simulink model "Teensy41_DC_motor_SysId"  (R2025b)
settings: Solver=FixedStepAuto  StartTime=0.0  StopTime=12  RelTol=1e-3  EnableMultiTasking=on
InitFcn:
  | run('Teensy41_system_init.m');
StopFcn:
  | run('Teensy41_to_save_data.m');
values from neighbouring files (symbols this model uses):
  ts = time(2)    [DC_Motor_SysId.m]    (also in DC_Motor_SysId_solve.m)
libraries: arduinolib x22
settings Model: ExtModeTrigDuration=2  Creator=ricardoaguilera  LastModifiedBy=nathan
settings SolverCC: AutoInsertRateTranBlk=on
settings OptimizationCC: EnhancedBackFolding=on  PassReuseOutputArgsAs=Individual arguments  ZeroExternalMemoryAtStartup=off  ZeroInternalMemoryAtStartup=off  MaxStackSize=64  OptimizeBlockOrder=speed  DifferentSizesBufferReuse=on  OptimizationCustomize=off  EfficientTunableParamExpr=on
settings DebuggingCC: ParameterTunabilityLossMsg=error
settings HardwareCC: ProdBitPerPointer=32.0  ProdBitPerSizeT=32.0  ProdBitPerPtrDiffT=32.0  ProdLargestAtomicInteger=Long  ProdLargestAtomicFloat=Double  ProdWordSize=32.0  ProdHWDeviceType=ARM Compatible->ARM Cortex
settings SFSimCC: MATLABDynamicMemAlloc=off
settings RTWCC: SystemTargetFile=ert.tlc  HardwareBoard=Teensy 4.1 (Arduino Compatible)  TemplateMakefile=ert_default_tmf  Toolchain=Arduino ARM M7  BuildConfiguration=Faster Runs  Description=Embedded Coder
settings CodeAppCC: ForceParamTrailComments=on  IgnoreCustomStorageClasses=off  OperatorAnnotations=on  SimulinkDataObjDesc=on  SFDataObjDesc=on  InsertBlockDesc=on
settings ERTTargetCC: ExtModeTransport=3.0  ExtModeStaticAlloc=on  ExtModeAutomaticAllocSize=off  ExtModeStaticAllocSize=65536.0  ExtModeMexFile=ext_xcp  ExtModeIntrfLevel=Level2 - Open  InlinedParameterPlacement=Hierarchical  SupportContinuousTime=on  SupportVariableSizeSignals=on

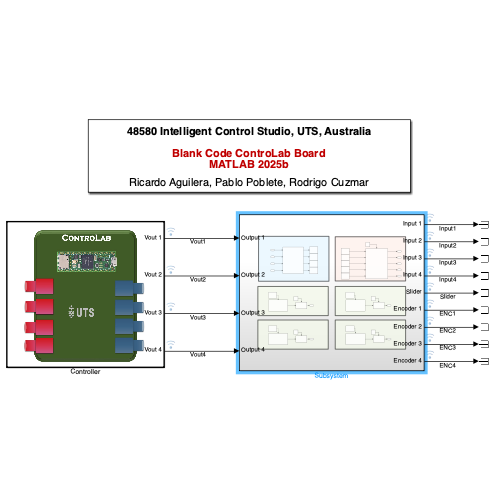
[thumbnail: Simulink's stored preview of the top-level diagram]
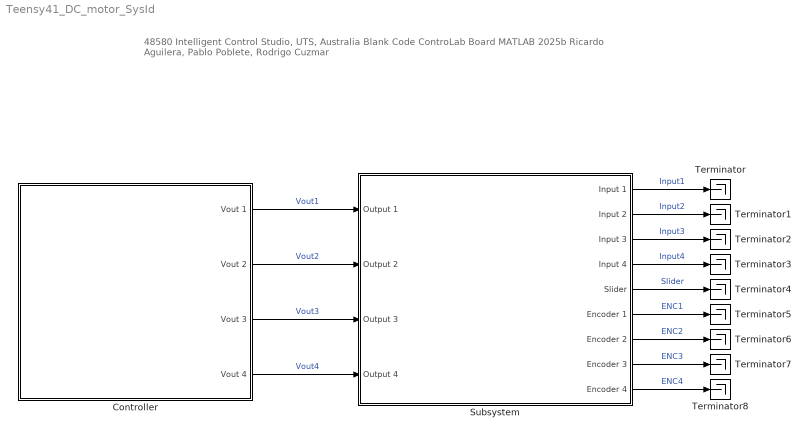
== system Teensy41_DC_motor_SysId ==
  note: 48580 Intelligent Control Studio, UTS, Australia
      |
      | Blank Code ControLab Board
      | MATLAB 2025b
      |
      | Ricardo Aguilera, Pablo Poblete, Rodrigo Cuzmar
  Controller : Subsystem  TreatAsAtomicUnit=on
      mask Display: image('Board_1.png');
  Subsystem : Subsystem
  Terminator{,1..8} (9 alike) : Terminator
  wires:
  Subsystem/8(Encoder 3) -> Terminator7/1  "ENC3"
  Subsystem/7(Encoder 2) -> Terminator6/1  "ENC2"
  Controller/3(Vout 3) -> Subsystem/3(Output 3)  "Vout3"
  Controller/4(Vout 4) -> Subsystem/4(Output 4)  "Vout4"
  Controller/2(Vout 2) -> Subsystem/2(Output 2)  "Vout2"
  Subsystem/5(Slider) -> Terminator4/1  "Slider"
  Subsystem/1(Input 1) -> Terminator/1  "Input1"
  Subsystem/9(Encoder 4) -> Terminator8/1  "ENC4"
  Subsystem/4(Input 4) -> Terminator3/1  "Input4"
  Subsystem/2(Input 2) -> Terminator1/1  "Input2"
  Subsystem/3(Input 3) -> Terminator2/1  "Input3"
  Subsystem/6(Encoder 1) -> Terminator5/1  "ENC1"
  Controller/1(Vout 1) -> Subsystem/1(Output 1)  "Vout1"

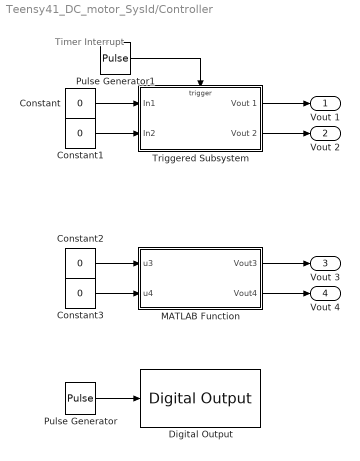
== system Teensy41_DC_motor_SysId/Controller ==
  note: Timer
      | Interrupt
  Constant{,1..3} (4 alike) : Constant  Value=0
  Digital Output : arduinolib/Digital Output  pinNumber=13  Direction=output  blockPlatform=arduino
  MATLAB Function : MATLAB Function  TreatAsAtomicUnit=on  SystemSampleTime=ts
  Pulse Generator : DiscretePulseGenerator  PulseType=Time based  Period=4  PulseWidth=50
  Pulse Generator1 : DiscretePulseGenerator  PulseType=Time based  Period=ts  PulseWidth=50
  Triggered Subsystem : Subsystem  TreatAsAtomicUnit=on
  Vout 1 : Outport
  Vout 2 : Outport  Port=2
  Vout 3 : Outport  Port=3
  Vout 4 : Outport  Port=4
  wires:
  Pulse Generator/1 -> Digital Output/1
  Triggered Subsystem/1(Vout 1) -> Vout 1/1
  Pulse Generator1/1 -> Triggered Subsystem/Trigger
  Constant/1 -> Triggered Subsystem/1(In1)
  MATLAB Function/2(Vout4) -> Vout 4/1
  MATLAB Function/1(Vout3) -> Vout 3/1
  Triggered Subsystem/2(Vout 2) -> Vout 2/1
  Constant1/1 -> Triggered Subsystem/2(In2)
  Constant2/1 -> MATLAB Function/1(u3)
  Constant3/1 -> MATLAB Function/2(u4)

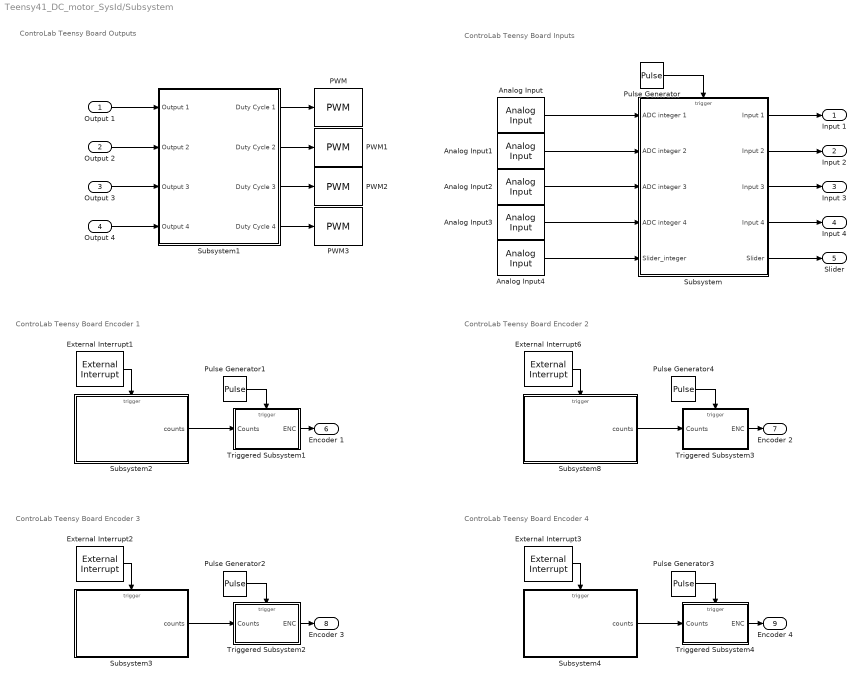
== system Teensy41_DC_motor_SysId/Subsystem ==
  note: ControLab Teensy Board Outputs
  note: ControLab Teensy Board Inputs
  note: ControLab Teensy Board Encoder 2
  note: ControLab Teensy Board Encoder 1
  note: ControLab Teensy Board Encoder 3
  note: ControLab Teensy Board Encoder 4
  Output 1 : Inport
  Output 2 : Inport  Port=2
  Output 3 : Inport  Port=3
  Output 4 : Inport  Port=4
  Analog Input : arduinolib/Analog Input  pinNumber=2  ReadResultsOnly=off  ConversionTriggerSource=Software  ExternalTriggerType=uint32( 0 )  OutputDataType=uint16  EnableConversionCompleteNotify=off  EnableOuputStatus=off  SampleTime=-1  blockPlatform=arduino
  Analog Input1 : arduinolib/Analog Input  pinNumber=3  ReadResultsOnly=off  ConversionTriggerSource=Software  ExternalTriggerType=uint32( 0 )  OutputDataType=uint16  EnableConversionCompleteNotify=off  EnableOuputStatus=off  SampleTime=-1  blockPlatform=arduino
  Analog Input2 : arduinolib/Analog Input  pinNumber=6  ReadResultsOnly=off  ConversionTriggerSource=Software  ExternalTriggerType=uint32( 0 )  OutputDataType=uint16  EnableConversionCompleteNotify=off  EnableOuputStatus=off  SampleTime=-1  blockPlatform=arduino
  Analog Input3 : arduinolib/Analog Input  pinNumber=7  ReadResultsOnly=off  ConversionTriggerSource=Software  ExternalTriggerType=uint32( 0 )  OutputDataType=uint16  EnableConversionCompleteNotify=off  EnableOuputStatus=off  SampleTime=-1  blockPlatform=arduino
  Analog Input4 : arduinolib/Analog Input  pinNumber=1  ReadResultsOnly=off  ConversionTriggerSource=Software  ExternalTriggerType=uint32( 0 )  OutputDataType=uint16  EnableConversionCompleteNotify=off  EnableOuputStatus=off  SampleTime=-1  blockPlatform=arduino
  External Interrupt1 : arduinolib/External Interrupt  Pin=40  PullUp=off  Mode=CHANGE  InterruptSimulationInput=off
  External Interrupt2 : arduinolib/External Interrupt  Pin=26  PullUp=off  Mode=CHANGE  InterruptSimulationInput=off
  External Interrupt3 : arduinolib/External Interrupt  Pin=30  PullUp=off  Mode=CHANGE  InterruptSimulationInput=off
  External Interrupt6 : arduinolib/External Interrupt  Pin=36  PullUp=off  Mode=CHANGE  InterruptSimulationInput=off
  PWM : arduinolib/PWM  pinNumber=2  frequencyType=Specify  desiredFrequency=4000  achievableFrequency=4000
  PWM1 : arduinolib/PWM  pinNumber=4  frequencyType=Specify  desiredFrequency=4000  achievableFrequency=4000
  PWM2 : arduinolib/PWM  pinNumber=5  frequencyType=Specify  desiredFrequency=4000  achievableFrequency=4000
  PWM3 : arduinolib/PWM  pinNumber=6  frequencyType=Specify  desiredFrequency=4000  achievableFrequency=4000
  Pulse Generator{,1..4} (5 alike) : DiscretePulseGenerator  PulseType=Time based  Period=ts  PulseWidth=50
  Subsystem : Subsystem
  Subsystem1 : Subsystem
  Subsystem2 : Subsystem
  Subsystem3 : Subsystem
  Subsystem4 : Subsystem
  Subsystem8 : Subsystem
  Triggered Subsystem1 : Subsystem  TreatAsAtomicUnit=on
  Triggered Subsystem2 : Subsystem  TreatAsAtomicUnit=on
  Triggered Subsystem3 : Subsystem  TreatAsAtomicUnit=on
  Triggered Subsystem4 : Subsystem  TreatAsAtomicUnit=on
  Input 1 : Outport
  Input 2 : Outport  Port=2
  Input 3 : Outport  Port=3
  Input 4 : Outport  Port=4
  Slider : Outport  Port=5
  Encoder 1 : Outport  Port=6
  Encoder 2 : Outport  Port=7
  Encoder 3 : Outport  Port=8
  Encoder 4 : Outport  Port=9
  wires:
  Pulse Generator/1 -> Subsystem/Trigger
  Analog Input/1 -> Subsystem/1(ADC integer 1)
  Analog Input1/1 -> Subsystem/2(ADC integer 2)
  Analog Input2/1 -> Subsystem/3(ADC integer 3)
  Analog Input3/1 -> Subsystem/4(ADC integer 4)
  Analog Input4/1 -> Subsystem/5(Slider_integer)
  Subsystem/1(Input 1) -> Input 1/1
  Subsystem/2(Input 2) -> Input 2/1
  Subsystem/3(Input 3) -> Input 3/1
  Subsystem/4(Input 4) -> Input 4/1
  Subsystem1/1(Duty Cycle 1) -> PWM/1
  Subsystem1/2(Duty Cycle 2) -> PWM1/1
  Subsystem1/3(Duty Cycle 3) -> PWM2/1
  Subsystem1/4(Duty Cycle 4) -> PWM3/1
  Output 1/1 -> Subsystem1/1(Output 1)
  Output 4/1 -> Subsystem1/4(Output 4)
  Output 3/1 -> Subsystem1/3(Output 3)
  Output 2/1 -> Subsystem1/2(Output 2)
  Subsystem/5(Slider) -> Slider/1
  Subsystem8/1(counts) -> Triggered Subsystem3/1(Counts)
  Pulse Generator4/1 -> Triggered Subsystem3/Trigger
  Triggered Subsystem3/1(ENC) -> Encoder 2/1
  External Interrupt6/1 -> Subsystem8/Trigger
  External Interrupt1/1 -> Subsystem2/Trigger
  Triggered Subsystem1/1(ENC) -> Encoder 1/1
  Pulse Generator1/1 -> Triggered Subsystem1/Trigger
  Subsystem2/1(counts) -> Triggered Subsystem1/1(Counts)
  Subsystem3/1(counts) -> Triggered Subsystem2/1(Counts)
  Pulse Generator2/1 -> Triggered Subsystem2/Trigger
  Triggered Subsystem2/1(ENC) -> Encoder 3/1
  External Interrupt2/1 -> Subsystem3/Trigger
  External Interrupt3/1 -> Subsystem4/Trigger
  Triggered Subsystem4/1(ENC) -> Encoder 4/1
  Pulse Generator3/1 -> Triggered Subsystem4/Trigger
  Subsystem4/1(counts) -> Triggered Subsystem4/1(Counts)

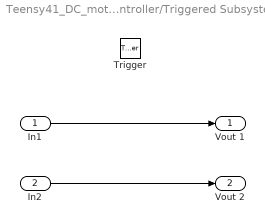
== system Teensy41_DC_motor_SysId/Controller/Triggered Subsystem ==
  In1 : Inport
  In2 : Inport  Port=2
  Trigger : TriggerPort  VariantControl=(inherit)
  Vout 1 : Outport
  Vout 2 : Outport  Port=2
  wires:
  In1/1 -> Vout 1/1
  In2/1 -> Vout 2/1

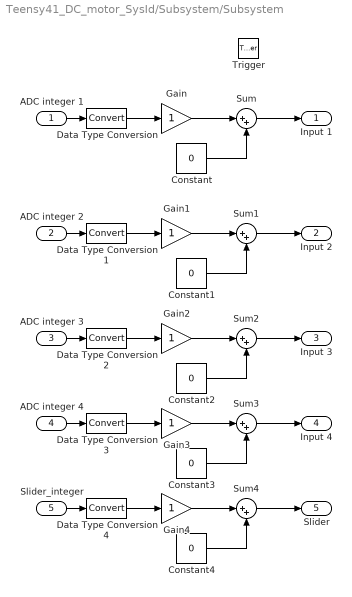
== system Teensy41_DC_motor_SysId/Subsystem/Subsystem ==
  ADC integer 1 : Inport
  ADC integer 2 : Inport  Port=2
  ADC integer 3 : Inport  Port=3
  ADC integer 4 : Inport  Port=4
  Slider_integer : Inport  Port=5
  Trigger : TriggerPort  VariantControl=(inherit)  PortDimensions=1
  Constant{,1..4} (5 alike) : Constant  Value=0
  Data Type Conversion{,1..4} (5 alike) : DataTypeConversion  SaturateOnIntegerOverflow=off  RndMeth=Floor
  Gain{,1..4} (5 alike) : Gain
  Sum{,1..4} (5 alike) : Sum  Inputs=|++
  Input 1 : Outport
  Input 2 : Outport  Port=2
  Input 3 : Outport  Port=3
  Input 4 : Outport  Port=4
  Slider : Outport  Port=5
  wires:
  ADC integer 1/1 -> Data Type Conversion/1
  Data Type Conversion/1 -> Gain/1
  Gain/1 -> Sum/1
  Constant/1 -> Sum/2
  Sum/1 -> Input 1/1
  Data Type Conversion1/1 -> Gain1/1
  Sum1/1 -> Input 2/1
  ADC integer 2/1 -> Data Type Conversion1/1
  Constant1/1 -> Sum1/2
  Gain1/1 -> Sum1/1
  Data Type Conversion2/1 -> Gain2/1
  Sum2/1 -> Input 3/1
  ADC integer 3/1 -> Data Type Conversion2/1
  Constant2/1 -> Sum2/2
  Gain2/1 -> Sum2/1
  Data Type Conversion3/1 -> Gain3/1
  Sum3/1 -> Input 4/1
  ADC integer 4/1 -> Data Type Conversion3/1
  Constant3/1 -> Sum3/2
  Gain3/1 -> Sum3/1
  Slider_integer/1 -> Data Type Conversion4/1
  Data Type Conversion4/1 -> Gain4/1
  Gain4/1 -> Sum4/1
  Constant4/1 -> Sum4/2
  Sum4/1 -> Slider/1

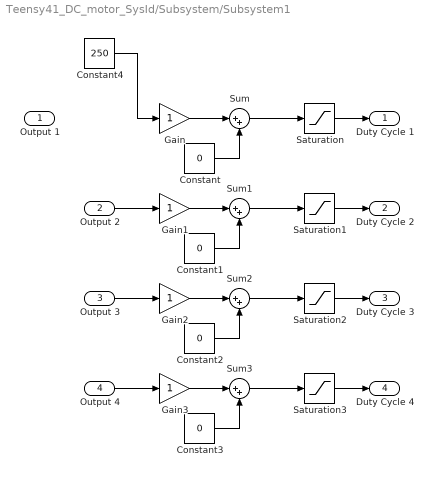
== system Teensy41_DC_motor_SysId/Subsystem/Subsystem1 ==
  Output 1 : Inport
  Output 2 : Inport  Port=2
  Output 3 : Inport  Port=3
  Output 4 : Inport  Port=4
  Constant{,1..3} (4 alike) : Constant  Value=0
  Constant4 : Constant  Value=250
  Gain{,1..3} (4 alike) : Gain
  Saturation{,1..3} (4 alike) : Saturate  UpperLimit=255  LowerLimit=1
  Sum{,1..3} (4 alike) : Sum  Inputs=|++
  Duty Cycle 1 : Outport
  Duty Cycle 2 : Outport  Port=2
  Duty Cycle 3 : Outport  Port=3
  Duty Cycle 4 : Outport  Port=4
  wires:
  Saturation/1 -> Duty Cycle 1/1
  Sum/1 -> Saturation/1
  Gain/1 -> Sum/1
  Constant/1 -> Sum/2
  Constant1/1 -> Sum1/2
  Gain1/1 -> Sum1/1
  Sum1/1 -> Saturation1/1
  Output 2/1 -> Gain1/1
  Saturation1/1 -> Duty Cycle 2/1
  Saturation2/1 -> Duty Cycle 3/1
  Output 3/1 -> Gain2/1
  Sum2/1 -> Saturation2/1
  Gain2/1 -> Sum2/1
  Constant2/1 -> Sum2/2
  Constant3/1 -> Sum3/2
  Gain3/1 -> Sum3/1
  Sum3/1 -> Saturation3/1
  Output 4/1 -> Gain3/1
  Saturation3/1 -> Duty Cycle 4/1
  Constant4/1 -> Gain/1

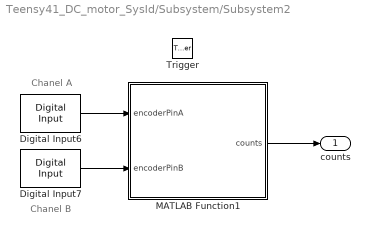
== system Teensy41_DC_motor_SysId/Subsystem/Subsystem2 ==
  note: Chanel B
  note: Chanel A
  Trigger : TriggerPort  TriggerType=function-call  VariantControl=(inherit)  PortDimensions=1
  Digital Input6 : arduinolib/Digital Input  pinNumber=39  mode=Default  Direction=input  SampleTime=-1  blockPlatform=arduino
  Digital Input7 : arduinolib/Digital Input  pinNumber=37  mode=Default  Direction=input  SampleTime=-1  blockPlatform=arduino
  MATLAB Function1 : MATLAB Function  TreatAsAtomicUnit=on
  counts : Outport
  wires:
  Digital Input7/1 -> MATLAB Function1/2(encoderPinB)
  Digital Input6/1 -> MATLAB Function1/1(encoderPinA)
  MATLAB Function1/1(counts) -> counts/1

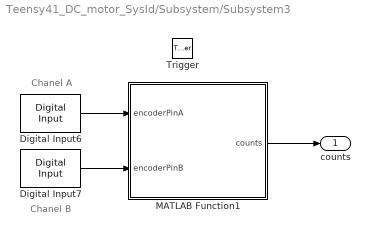
== system Teensy41_DC_motor_SysId/Subsystem/Subsystem3 ==
  note: Chanel A
  note: Chanel B
  Trigger : TriggerPort  TriggerType=function-call  VariantControl=(inherit)  PortDimensions=1
  Digital Input6 : arduinolib/Digital Input  pinNumber=25  mode=Default  Direction=input  SampleTime=-1  blockPlatform=arduino
  Digital Input7 : arduinolib/Digital Input  pinNumber=27  mode=Default  Direction=input  SampleTime=-1  blockPlatform=arduino
  MATLAB Function1 : MATLAB Function  TreatAsAtomicUnit=on
  counts : Outport
  wires:
  MATLAB Function1/1(counts) -> counts/1
  Digital Input6/1 -> MATLAB Function1/1(encoderPinA)
  Digital Input7/1 -> MATLAB Function1/2(encoderPinB)

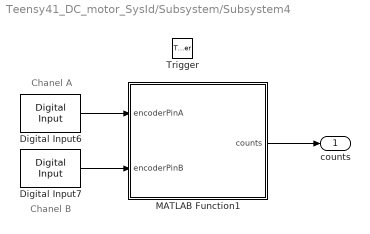
== system Teensy41_DC_motor_SysId/Subsystem/Subsystem4 ==
  note: Chanel B
  note: Chanel A
  Trigger : TriggerPort  TriggerType=function-call  VariantControl=(inherit)  PortDimensions=1
  Digital Input6 : arduinolib/Digital Input  pinNumber=29  mode=Default  Direction=input  SampleTime=-1  blockPlatform=arduino
  Digital Input7 : arduinolib/Digital Input  pinNumber=31  mode=Default  Direction=input  SampleTime=-1  blockPlatform=arduino
  MATLAB Function1 : MATLAB Function  TreatAsAtomicUnit=on
  counts : Outport
  wires:
  Digital Input7/1 -> MATLAB Function1/2(encoderPinB)
  Digital Input6/1 -> MATLAB Function1/1(encoderPinA)
  MATLAB Function1/1(counts) -> counts/1

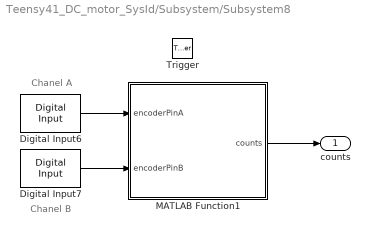
== system Teensy41_DC_motor_SysId/Subsystem/Subsystem8 ==
  note: Chanel A
  note: Chanel B
  Trigger : TriggerPort  TriggerType=function-call  VariantControl=(inherit)  PortDimensions=1
  Digital Input6 : arduinolib/Digital Input  pinNumber=35  mode=Default  Direction=input  SampleTime=-1  blockPlatform=arduino
  Digital Input7 : arduinolib/Digital Input  pinNumber=33  mode=Default  Direction=input  SampleTime=-1  blockPlatform=arduino
  MATLAB Function1 : MATLAB Function  TreatAsAtomicUnit=on
  counts : Outport
  wires:
  MATLAB Function1/1(counts) -> counts/1
  Digital Input6/1 -> MATLAB Function1/1(encoderPinA)
  Digital Input7/1 -> MATLAB Function1/2(encoderPinB)

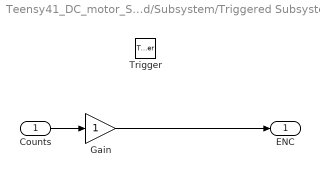
== system Teensy41_DC_motor_SysId/Subsystem/Triggered Subsystem1 ==
  Counts : Inport
  Trigger : TriggerPort  VariantControl=(inherit)
  Gain : Gain
  ENC : Outport
  wires:
  Gain/1 -> ENC/1
  Counts/1 -> Gain/1

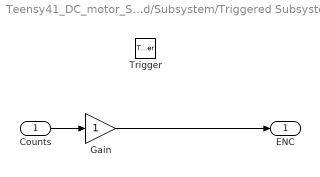
== system Teensy41_DC_motor_SysId/Subsystem/Triggered Subsystem2 ==
  Counts : Inport
  Trigger : TriggerPort  VariantControl=(inherit)
  Gain : Gain
  ENC : Outport
  wires:
  Counts/1 -> Gain/1
  Gain/1 -> ENC/1

== system Teensy41_DC_motor_SysId/Subsystem/Triggered Subsystem3 ==
  Counts : Inport
  Trigger : TriggerPort  VariantControl=(inherit)
  Gain : Gain
  ENC : Outport
  wires:
  Counts/1 -> Gain/1
  Gain/1 -> ENC/1

== system Teensy41_DC_motor_SysId/Subsystem/Triggered Subsystem4 ==
  Counts : Inport
  Trigger : TriggerPort  VariantControl=(inherit)
  Gain : Gain
  ENC : Outport
  wires:
  Gain/1 -> ENC/1
  Counts/1 -> Gain/1

== matlab function Teensy41_DC_motor_SysId/Controller/MATLAB Function ==
  data: u3 input; Vout3 output; u4 input; Vout4 output
function [Vout3, Vout4]  = fcn(u3, u4)

Vout3 = u3;
Vout4 = u4;

end

== matlab function Teensy41_DC_motor_SysId/Subsystem/Subsystem3/MATLAB Function1 ==
  data: counts output; encoderPinA input; encoderPinB input
function counts = computeEncoderPosition(encoderPinA, encoderPinB)
% This function determines the motor position based on the latest 
% state update for the encoder digital inputs. 

%% Persistent variables to store previous states and position
persistent lastPosition

% Initialize persistent variables on the first run
if isempty(lastPosition)

    lastPosition = 0;
end


%% Determine direction and update position
if (encoderPinA == encoderPinB)
    % Direction is forward
    lastPosition = lastPosition + 1;
else
    % Direction is backward
    lastPosition = lastPosition - 1;
end

%% Output the current position
counts = lastPosition;

== matlab function Teensy41_DC_motor_SysId/Subsystem/Subsystem4/MATLAB Function1 ==
  data: counts output; encoderPinA input; encoderPinB input
function counts = computeEncoderPosition(encoderPinA, encoderPinB)
% This function determines the motor position based on the latest 
% state update for the encoder digital inputs. 

%% Persistent variables to store previous states and position
persistent lastPosition

% Initialize persistent variables on the first run
if isempty(lastPosition)

    lastPosition = 0;
end


%% Determine direction and update position
if (encoderPinA == encoderPinB)
    % Direction is forward
    lastPosition = lastPosition + 1;
else
    % Direction is backward
    lastPosition = lastPosition - 1;
end

%% Output the current position
counts = lastPosition;

== matlab function Teensy41_DC_motor_SysId/Subsystem/Subsystem8/MATLAB Function1 ==
  data: counts output; encoderPinA input; encoderPinB input
function counts = computeEncoderPosition(encoderPinA, encoderPinB)
% This function determines the motor position based on the latest 
% state update for the encoder digital inputs. 

%% Persistent variables to store previous states and position
persistent lastPosition

% Initialize persistent variables on the first run
if isempty(lastPosition)

    lastPosition = 0;
end


%% Determine direction and update position
if (encoderPinA == encoderPinB)
    % Direction is forward
    lastPosition = lastPosition + 1;
else
    % Direction is backward
    lastPosition = lastPosition - 1;
end

%% Output the current position
counts = lastPosition;

== matlab function Teensy41_DC_motor_SysId/Subsystem/Subsystem2/MATLAB Function1 ==
  data: counts output; encoderPinA input; encoderPinB input
function counts = computeEncoderPosition(encoderPinA, encoderPinB)
% This function determines the motor position based on the latest 
% state update for the encoder digital inputs. 

%% Persistent variables to store previous states and position
persistent lastPosition

% Initialize persistent variables on the first run
if isempty(lastPosition)

    lastPosition = 0;
end


%% Determine direction and update position
if (encoderPinA == encoderPinB)
    % Direction is forward
    lastPosition = lastPosition + 1;
else
    % Direction is backward
    lastPosition = lastPosition - 1;
end

%% Output the current position
counts = lastPosition;
